simulink model "num1"  (R2019a)
settings: Solver=VariableStepAuto  StartTime=0.0  StopTime=10.0  RelTol=1e-3
settings Model: Creator=julia  LastModifiedBy=julia

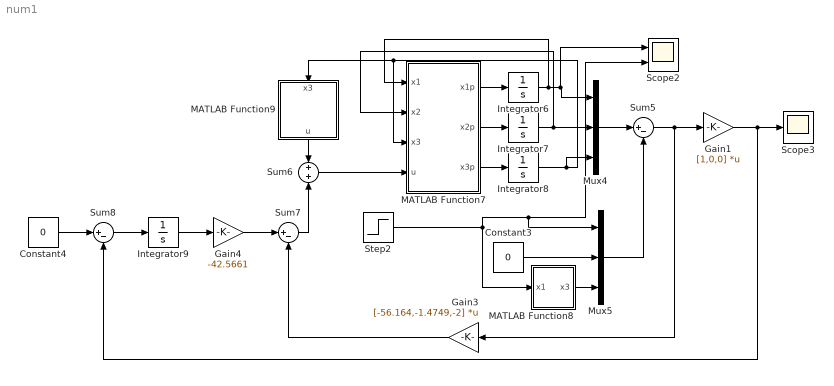
== system num1 ==
  Constant3 : Constant  Value=0
  Constant4 : Constant  Value=0
  Gain1 : Gain  Gain=[1,0,0]  Multiplication=Matrix(K*u)
  Gain3 : Gain  Gain=[-56.164,-1.4749,-2]  Multiplication=Matrix(K*u)
  Gain4 : Gain  Gain=-42.5661
  Integrator6 : Integrator  InitialCondition=5e-3
  Integrator7 : Integrator
  Integrator8 : Integrator  InitialCondition=0.070035
  Integrator9 : Integrator
  MATLAB Function7 : MATLAB Function  TreatAsAtomicUnit=on
  MATLAB Function8 : MATLAB Function  TreatAsAtomicUnit=on
  MATLAB Function9 : MATLAB Function  TreatAsAtomicUnit=on
  Mux4 : Mux  Inputs=3
  Mux5 : Mux  Inputs=3
  Scope2 : Scope  NumInputPorts=2
  Scope3 : Scope
  Step2 : Step  Time=0  Before=5e-3  After=10e-3  SampleTime=0
  Sum5 : Sum  Inputs=|+-
  Sum6 : Sum  Inputs=+|+
  Sum7 : Sum  Inputs=|+-
  Sum8 : Sum  Inputs=|+-
  wires:
  Gain3/1 -> Sum7/2
  Integrator9/1 -> Gain4/1
  Constant4/1 -> Sum8/1
  Gain1/1 -> Sum8/2, Scope3/1
  Sum5/1 -> Gain1/1, Gain3/1
  Sum7/1 -> Sum6/2
  Sum8/1 -> Integrator9/1
  Gain4/1 -> Sum7/1
  MATLAB Function9/1(u) -> Sum6/1
  Sum6/1 -> MATLAB Function7/4(u)
  Mux5/1 -> Sum5/2
  MATLAB Function8/1(x3) -> Mux5/3
  Step2/1 -> MATLAB Function8/1(x1), Mux5/1, Scope2/2
  Constant3/1 -> Mux5/2
  Mux4/1 -> Sum5/1
  Integrator8/1 -> Mux4/3, MATLAB Function7/3(x3), MATLAB Function9/1(x3)
  Integrator7/1 -> Mux4/2, MATLAB Function7/2(x2)
  Integrator6/1 -> Mux4/1, Scope2/1, MATLAB Function7/1(x1)
  MATLAB Function7/3(x3p) -> Integrator8/1
  MATLAB Function7/2(x2p) -> Integrator7/1
  MATLAB Function7/1(x1p) -> Integrator6/1

== matlab function num1/MATLAB Function7 ==
  data: x1 input size=1; x1p output size=1; x2 input size=1; x3 input size=1; x2p output size=1; x3p output size=1; u input size=1
function [x1p,x2p,x3p] = planta(x1,x2,x3,u)
c=0.1;
m=0.01;
L=100e-3;
r=10;
g=9.81;

x1p=x2;
x2p=g-(c/m)*((x3^2)/x1);
x3p=-(r/L)*x3+(1/L)*u;

== matlab function num1/MATLAB Function8 ==
  data: x1 input size=1; x3 output size=1
function x3  = fcn(x1)
c=1
m=0.1
L=0.01
r=1
g=9.81

x3=sqrt((m*g*x1)/c);

== matlab function num1/MATLAB Function9 ==
  data: x3 input size=1; u output size=1
function u  = u(x3)
c=1
m=0.1
L=0.01
r=1
g=9.81

u=r*x3;
